simulink model "nmpc_blocks_2023a"  (R2023b)
settings: Solver=ode45  StartTime=0.0  StopTime=10  FixedStep=1  RelTol=1e-3  EnableMultiTasking=on
values from neighbouring files (symbols this model uses):
  K = nmpc_design_st2(par)    [es2.m]    (also in nmpc_design_template.m)
settings Model: Creator=carlonovara  LastModifiedBy=carlonovara
settings SolverCC: AlgebraicLoopSolver=TrustRegion  AutoInsertRateTranBlk=on
settings DataIOCC: ReturnWorkspaceOutputs=off
settings OptimizationCC: LifeSpan=inf
settings DebuggingCC: UnconnectedInputMsg=warning  UnconnectedOutputMsg=warning  UnconnectedLineMsg=warning  SFUnexpectedBacktrackingDiag=warning  SFNoUnconditionalDefaultTransitionDiag=warning  SFExecutionAtInitializationDiag=none  ArithmeticOperatorsInVariantConditions=warning
settings HardwareCC: ProdBitPerSizeT=32  ProdBitPerPtrDiffT=32  ProdWordSize=32  ProdHWDeviceType=Specified
settings ModelReferenceCC: EnableRefExpFcnMdlSchedulingChecks=on
settings SFSimCC: SimUseLocalCustomCode=off  CustomCodeUndefinedFunction=UseInterfaceOnly
settings RTWCC: RTWUseLocalCustomCode=off  DLArmComputeVersion=19.05
settings CodeAppCC: StateflowObjectComments=on
settings GRTTargetCC: TargetLangStandard=C89/C90 (ANSI)
settings ConfigComp: CovMetricSettings=dw  CovSaveCumulativeToWorkspaceVar=on  CovSaveSingleToWorkspaceVar=on  CovExternalEMLEnable=off

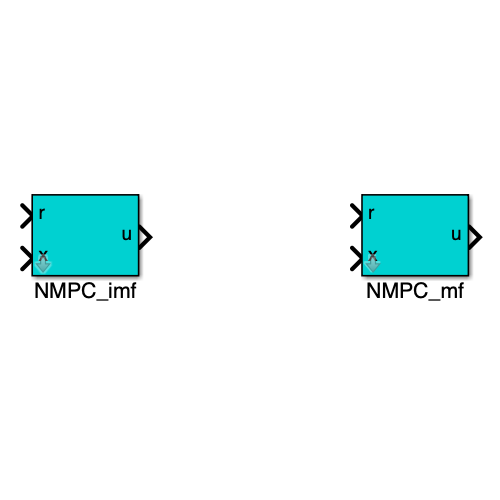
[thumbnail: Simulink's stored preview of the top-level diagram]
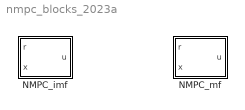
== system nmpc_blocks_2023a ==
  NMPC_imf : Subsystem  mask{K=K}
      mask prompts: K "NMPC structure"
  NMPC_mf : Subsystem  mask{K=K}
      mask prompts: K "NMPC structure"

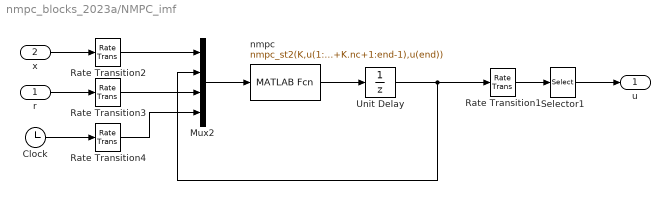
== system nmpc_blocks_2023a/NMPC_imf ==
  r : Inport
  x : Inport  Port=2
  Clock : Clock
  Mux2 : Mux
  Rate Transition{1..4} (4 alike) : RateTransition  OutPortSampleTime=K.Ts
  Selector1 : Selector  InputPortWidth=K.nc  IndexOptions=Index vector (dialog)  Indices=1:K.nu  OutputSizes=1
  Unit Delay : UnitDelay  InitialCondition=zeros(K.nc,1)  SampleTime=K.Ts  HasFrameUpgradeWarning=on
  nmpc : MATLABFcn  MATLABFcn=nmpc_st2(K,u(1:K.nx),u(K.nx+1:K.nx+K.nc),u(K.nx+K.nc+1:end-1),u(end))  OutputDimensions=K.nc
  u : Outport  PortDimensions=K.nu
  wires:
  x/1 -> Rate Transition2/1
  Unit Delay/1 -> Rate Transition1/1, Mux2/2
  Mux2/1 -> nmpc/1
  r/1 -> Rate Transition3/1
  Rate Transition2/1 -> Mux2/1
  Rate Transition1/1 -> Selector1/1
  Rate Transition3/1 -> Mux2/3
  nmpc/1 -> Unit Delay/1
  Selector1/1 -> u/1
  Clock/1 -> Rate Transition4/1
  Rate Transition4/1 -> Mux2/4

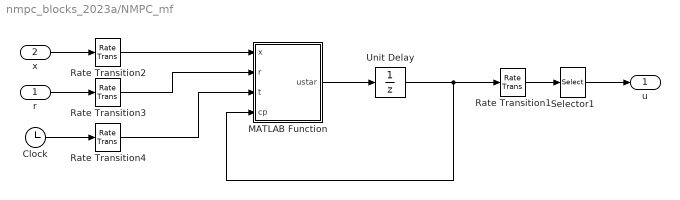
== system nmpc_blocks_2023a/NMPC_mf ==
  r : Inport
  x : Inport  Port=2
  Clock : Clock
  MATLAB Function : MATLAB Function  TreatAsAtomicUnit=on
  Rate Transition{1..4} (4 alike) : RateTransition  OutPortSampleTime=K.Ts
  Selector1 : Selector  InputPortWidth=K.nc  IndexOptions=Index vector (dialog)  Indices=1:K.nu  OutputSizes=1
  Unit Delay : UnitDelay  InitialCondition=zeros(K.nc,1)  SampleTime=K.Ts  HasFrameUpgradeWarning=on
  u : Outport  PortDimensions=K.nu
  wires:
  Rate Transition4/1 -> MATLAB Function/3(t)
  Clock/1 -> Rate Transition4/1
  Selector1/1 -> u/1
  MATLAB Function/1(ustar) -> Unit Delay/1
  Rate Transition3/1 -> MATLAB Function/2(r)
  Rate Transition1/1 -> Selector1/1
  Rate Transition2/1 -> MATLAB Function/1(x)
  r/1 -> Rate Transition3/1
  Unit Delay/1 -> Rate Transition1/1, MATLAB Function/4(cp)
  x/1 -> Rate Transition2/1

== matlab function nmpc_blocks_2023a/NMPC_mf/MATLAB Function ==
  data: K parameter; x input; ustar output; r input; t input; cp input
function ustar=fcn(K,x,r,t,cp)

ustar=nmpc_st2(K,x,cp,r,t);
